simulink library "AircraftStateFromPositions"  (R2018b)
settings: Solver=VariableStepAuto  StartTime=0.0  StopTime=10.0  RelTol=1e-3
libraries: simulink x3
settings Model: Creator=BI28030  LastModifiedBy=BI28030

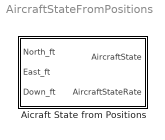
== system AircraftStateFromPositions ==
  Aicraft State from Positions : Subsystem  mask(Aircraft State from Positions){}
      mask help: Create an aircraft state bus from position signals
      mask Help:
      | Create an aircraft state bus from position signals
      | 
      | Speed and heading are set using first order difference on input positions.
      | All other quantities are set to zero.

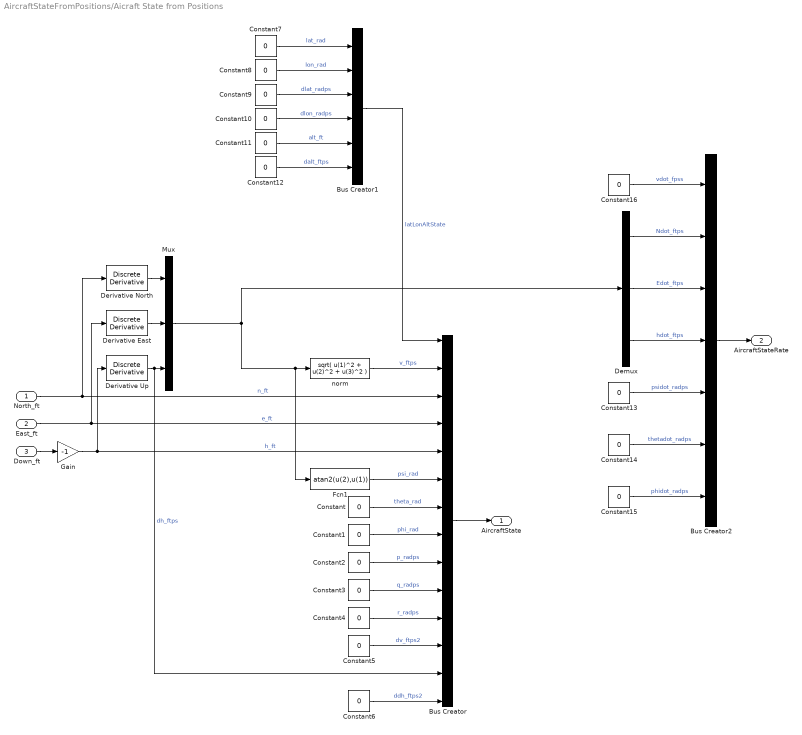
== system AircraftStateFromPositions/Aicraft State from Positions ==
  North_ft : Inport
  East_ft : Inport  Port=2
  Down_ft : Inport  Port=3
  Bus Creator : BusCreator  Inputs=14
  Bus Creator1 : BusCreator  Inputs=6  OutDataTypeStr=Bus: LatLonAltMeasurement
  Bus Creator2 : BusCreator  Inputs=7
  Constant{,1..16} (17 alike) : Constant  Value=0
  Demux : Demux  Outputs=3
  Derivative East : simulink/Discrete/Discrete Derivative  gainval=1.0  ICPrevScaledInput=0.0  OutMin=[]  OutMax=[]  OutDataType=fixdt(1, 16)  OutScaling=2^-10  DoSatur=off
  Derivative North : simulink/Discrete/Discrete Derivative  gainval=1.0  ICPrevScaledInput=0.0  OutMin=[]  OutMax=[]  OutDataType=fixdt(1, 16)  OutScaling=2^-10  DoSatur=off
  Derivative Up : simulink/Discrete/Discrete Derivative  gainval=1.0  ICPrevScaledInput=0.0  OutMin=[]  OutMax=[]  OutDataType=fixdt(1, 16)  OutScaling=2^-10  DoSatur=off
  Fcn1 : Fcn  Expr=atan2(u(2),u(1))
  Gain : Gain  Gain=-1
  Mux : Mux  Inputs=3
  norm : Fcn  Expr=sqrt( u(1)^2 + u(2)^2 + u(3)^2 )
  AircraftState : Outport  OutDataTypeStr=Bus: AircraftState
  AircraftStateRate : Outport  Port=2  OutDataTypeStr=Bus: AircraftStateRate
  wires:
  Bus Creator/1 -> AircraftState/1
  Bus Creator1/1 -> Bus Creator/1  "latLonAltState"
  norm/1 -> Bus Creator/2  "v_ftps"
  North_ft/1 -> Derivative North/1, Bus Creator/3  "n_ft"
  East_ft/1 -> Derivative East/1, Bus Creator/4  "e_ft"
  Gain/1 -> Derivative Up/1, Bus Creator/5  "h_ft"
  Fcn1/1 -> Bus Creator/6  "psi_rad"
  Constant/1 -> Bus Creator/7  "theta_rad"
  Constant1/1 -> Bus Creator/8  "phi_rad"
  Constant2/1 -> Bus Creator/9  "p_radps"
  Constant3/1 -> Bus Creator/10  "q_radps"
  Constant4/1 -> Bus Creator/11  "r_radps"
  Constant5/1 -> Bus Creator/12  "dv_ftps2"
  Derivative Up/1 -> Bus Creator/13, Mux/3  "dh_ftps"
  Constant6/1 -> Bus Creator/14  "ddh_ftps2"
  Down_ft/1 -> Gain/1
  Derivative North/1 -> Mux/1
  Derivative East/1 -> Mux/2
  Constant7/1 -> Bus Creator1/1  "lat_rad"
  Constant8/1 -> Bus Creator1/2  "lon_rad"
  Constant9/1 -> Bus Creator1/3  "dlat_radps"
  Constant10/1 -> Bus Creator1/4  "dlon_radps"
  Constant11/1 -> Bus Creator1/5  "alt_ft"
  Constant12/1 -> Bus Creator1/6  "dalt_ftps"
  Mux/1 -> Demux/1, Fcn1/1, norm/1
  Bus Creator2/1 -> AircraftStateRate/1
  Constant16/1 -> Bus Creator2/1  "vdot_fpss"
  Demux/1 -> Bus Creator2/2  "Ndot_ftps"
  Demux/2 -> Bus Creator2/3  "Edot_ftps"
  Demux/3 -> Bus Creator2/4  "hdot_ftps"
  Constant13/1 -> Bus Creator2/5  "psidot_radps"
  Constant14/1 -> Bus Creator2/6  "thetadot_radps"
  Constant15/1 -> Bus Creator2/7  "phidot_radps"
